simulink model "rpoco16"  (R2013a)
settings: Solver=VariableStepDiscrete  SolverMode=SingleTasking  StartTime=0.0  StopTime=10.0  RelTol=1e-3
libraries: xbsIndex_r4 x7152, casper_library_misc x156, casper_library_multipliers x68, casper_library_sources x8, xps_library x5, casper_library_delays x1
(part 9 of 84)

== system rpoco16/xengine16_muxed/bj ==
  a+bi : Inport
  c+di : Inport  Port=2
  new_acc : Inport  Port=3
  Convert{,1..3} (4 alike) : xbsIndex_r4/Convert  gui_display_data_type=Fixed-point  arith_type="Signed  (2's comp)"  n_bits=16  bin_pt=15  float_type=Single  exp_bits=8  fraction_bits=24  quantization="Round  (unbiased: Even Values)"  overflow=Wrap  en=off  latency=0  dbl_ovrd=off  pipeline=off  block_type=convert
      settings: block_version=11.4
  Counter2 : xbsIndex_r4/Counter  cnt_type=Free Running  cnt_to=Inf  operation=Up  start_count=0  cnt_by_val=1  arith_type=Unsigned  n_bits=max(nchan+1,11)  bin_pt=0  load_pin=off  rst=on  en=on  explicit_period=on  period=1  dbl_ovrd=off  use_behavioral_HDL=off  implementation=Fabric  use_rpm=off  block_type=counter
  Delay1 : xbsIndex_r4/Delay  rst=off  infoeditControl=Selection of Reset will increase slice count due to use of real FFs and instead of SRLs  en=off  latency=mult_latency + add_latency  dbl_ovrd=off  reg_retiming=off  block_type=delay
  c_to_ri : casper_library_misc/c_to_ri  n_bits=n_bits  bin_pt=n_bits-1
  c_to_ri1 : casper_library_misc/c_to_ri  n_bits=n_bits  bin_pt=n_bits-1
  cmult_4bit_em* : casper_library_multipliers/cmult_4bit_em*  mult_latency=mult_latency  add_latency=add_latency
  imag : Subsystem  Tag=xps:bram  AncestorBlock=xps_library/Shared BRAM  mask{arith_type=Signed  (2's comp), addr_width=max(nchan+1,11), data_width=32, reg_prim_output=off, reg_core_output=off, optimization=Minimum_Area, data_bin_pt=min(2*(n_bits-1), 30), init_vals=0, sample_rate=1}
      mask prompts: arith_type "Output Data Type"; addr_width "Address width"; data_width "Data Width"; reg_prim_output "Register Primitive Output"; reg_core_output "Register Core Output"; data_bin_pt "Data Binary Point"; init_vals "Initial values (simulation only)"; sample_rate "Sample rate"
      mask init:
      | shared_bram_mask;
      mask TypeOptions arith_type: Unsigned | Signed  (2's comp)
      mask TypeOptions data_width: 8 | 16 | 32 | 64 | 128
      mask TypeOptions optimization: Minimum_Area | Low_Power
  real : Subsystem  Tag=xps:bram  AncestorBlock=xps_library/Shared BRAM  mask{arith_type=Signed  (2's comp), addr_width=max(nchan+1,11), data_width=32, reg_prim_output=off, reg_core_output=off, optimization=Minimum_Area, data_bin_pt=min(2*(n_bits-1), 30), init_vals=0, sample_rate=1}
      mask prompts: arith_type "Output Data Type"; addr_width "Address width"; data_width "Data Width"; reg_prim_output "Register Primitive Output"; reg_core_output "Register Core Output"; data_bin_pt "Data Binary Point"; init_vals "Initial values (simulation only)"; sample_rate "Sample rate"
      mask init:
      | shared_bram_mask;
      mask TypeOptions arith_type: Unsigned | Signed  (2's comp)
      mask TypeOptions data_width: 8 | 16 | 32 | 64 | 128
      mask TypeOptions optimization: Minimum_Area | Low_Power
  simple_bram_vacc : Subsystem  AncestorBlock=casper_library_accumulators/simple_bram_vacc  mask(simple_bram_vacc){vec_len=2048, arith_type=Signed, n_bits=32, bin_pt=30}
      mask prompts: vec_len "Vector length:"; arith_type "Output type:"; n_bits "Bit width (output):"; bin_pt "Binary point (output):"
      mask help: This simple vector accumulator is based on a shift register. It outputs its previous accumulated vector after a new_acc pulse is received.
      mask init:
      | simple_bram_vacc_init(gcb, ...
      |     'vec_len', vec_len, ...
      |     'arith_type', arith_type, ...
      |     'n_bits', n_bits, ...
      |     'bin_pt', bin_pt);
      mask TypeOptions arith_type: Signed | Unsigned
  simple_bram_vacc1 : Subsystem  AncestorBlock=casper_library_accumulators/simple_bram_vacc  mask(simple_bram_vacc){vec_len=2048, arith_type=Signed, n_bits=32, bin_pt=30}
      mask prompts: vec_len "Vector length:"; arith_type "Output type:"; n_bits "Bit width (output):"; bin_pt "Binary point (output):"
      mask help: This simple vector accumulator is based on a shift register. It outputs its previous accumulated vector after a new_acc pulse is received.
      mask init:
      | simple_bram_vacc_init(gcb, ...
      |     'vec_len', vec_len, ...
      |     'arith_type', arith_type, ...
      |     'n_bits', n_bits, ...
      |     'bin_pt', bin_pt);
      mask TypeOptions arith_type: Signed | Unsigned
  wires:
  Convert3/1 -> cmult_4bit_em*/4
  Convert2/1 -> cmult_4bit_em*/3
  Convert1/1 -> cmult_4bit_em*/2
  Convert/1 -> cmult_4bit_em*/1
  c_to_ri/1 -> Convert/1
  c_to_ri/2 -> Convert1/1
  c_to_ri1/1 -> Convert2/1
  c_to_ri1/2 -> Convert3/1
  a+bi/1 -> c_to_ri/1
  c+di/1 -> c_to_ri1/1
  new_acc/1 -> Delay1/1
  simple_bram_vacc/2(valid) -> Counter2/2, real/3(we)
  Counter2/1 -> real/1(addr), imag/1(addr)
  simple_bram_vacc/1(dout) -> real/2(data_in)
  Delay1/1 -> simple_bram_vacc1/1(new_acc), simple_bram_vacc/1(new_acc), Counter2/1
  simple_bram_vacc1/1(dout) -> imag/2(data_in)
  simple_bram_vacc1/2(valid) -> imag/3(we)
  cmult_4bit_em*/1 -> simple_bram_vacc/2(din)
  cmult_4bit_em*/2 -> simple_bram_vacc1/2(din)

== system rpoco16/xengine16_muxed/bk ==
  a+bi : Inport
  c+di : Inport  Port=2
  new_acc : Inport  Port=3
  Convert{,1..3} (4 alike) : xbsIndex_r4/Convert  gui_display_data_type=Fixed-point  arith_type="Signed  (2's comp)"  n_bits=16  bin_pt=15  float_type=Single  exp_bits=8  fraction_bits=24  quantization="Round  (unbiased: Even Values)"  overflow=Wrap  en=off  latency=0  dbl_ovrd=off  pipeline=off  block_type=convert
      settings: block_version=11.4
  Counter2 : xbsIndex_r4/Counter  cnt_type=Free Running  cnt_to=Inf  operation=Up  start_count=0  cnt_by_val=1  arith_type=Unsigned  n_bits=max(nchan+1,11)  bin_pt=0  load_pin=off  rst=on  en=on  explicit_period=on  period=1  dbl_ovrd=off  use_behavioral_HDL=off  implementation=Fabric  use_rpm=off  block_type=counter
  Delay1 : xbsIndex_r4/Delay  rst=off  infoeditControl=Selection of Reset will increase slice count due to use of real FFs and instead of SRLs  en=off  latency=mult_latency + add_latency  dbl_ovrd=off  reg_retiming=off  block_type=delay
  c_to_ri : casper_library_misc/c_to_ri  n_bits=n_bits  bin_pt=n_bits-1
  c_to_ri1 : casper_library_misc/c_to_ri  n_bits=n_bits  bin_pt=n_bits-1
  cmult_4bit_em* : casper_library_multipliers/cmult_4bit_em*  mult_latency=mult_latency  add_latency=add_latency
  imag : Subsystem  Tag=xps:bram  AncestorBlock=xps_library/Shared BRAM  mask{arith_type=Signed  (2's comp), addr_width=max(nchan+1,11), data_width=32, reg_prim_output=off, reg_core_output=off, optimization=Minimum_Area, data_bin_pt=min(2*(n_bits-1), 30), init_vals=0, sample_rate=1}
      mask prompts: arith_type "Output Data Type"; addr_width "Address width"; data_width "Data Width"; reg_prim_output "Register Primitive Output"; reg_core_output "Register Core Output"; data_bin_pt "Data Binary Point"; init_vals "Initial values (simulation only)"; sample_rate "Sample rate"
      mask init:
      | shared_bram_mask;
      mask TypeOptions arith_type: Unsigned | Signed  (2's comp)
      mask TypeOptions data_width: 8 | 16 | 32 | 64 | 128
      mask TypeOptions optimization: Minimum_Area | Low_Power
  real : Subsystem  Tag=xps:bram  AncestorBlock=xps_library/Shared BRAM  mask{arith_type=Signed  (2's comp), addr_width=max(nchan+1,11), data_width=32, reg_prim_output=off, reg_core_output=off, optimization=Minimum_Area, data_bin_pt=min(2*(n_bits-1), 30), init_vals=0, sample_rate=1}
      mask prompts: arith_type "Output Data Type"; addr_width "Address width"; data_width "Data Width"; reg_prim_output "Register Primitive Output"; reg_core_output "Register Core Output"; data_bin_pt "Data Binary Point"; init_vals "Initial values (simulation only)"; sample_rate "Sample rate"
      mask init:
      | shared_bram_mask;
      mask TypeOptions arith_type: Unsigned | Signed  (2's comp)
      mask TypeOptions data_width: 8 | 16 | 32 | 64 | 128
      mask TypeOptions optimization: Minimum_Area | Low_Power
  simple_bram_vacc : Subsystem  AncestorBlock=casper_library_accumulators/simple_bram_vacc  mask(simple_bram_vacc){vec_len=2048, arith_type=Signed, n_bits=32, bin_pt=30}
      mask prompts: vec_len "Vector length:"; arith_type "Output type:"; n_bits "Bit width (output):"; bin_pt "Binary point (output):"
      mask help: This simple vector accumulator is based on a shift register. It outputs its previous accumulated vector after a new_acc pulse is received.
      mask init:
      | simple_bram_vacc_init(gcb, ...
      |     'vec_len', vec_len, ...
      |     'arith_type', arith_type, ...
      |     'n_bits', n_bits, ...
      |     'bin_pt', bin_pt);
      mask TypeOptions arith_type: Signed | Unsigned
  simple_bram_vacc1 : Subsystem  AncestorBlock=casper_library_accumulators/simple_bram_vacc  mask(simple_bram_vacc){vec_len=2048, arith_type=Signed, n_bits=32, bin_pt=30}
      mask prompts: vec_len "Vector length:"; arith_type "Output type:"; n_bits "Bit width (output):"; bin_pt "Binary point (output):"
      mask help: This simple vector accumulator is based on a shift register. It outputs its previous accumulated vector after a new_acc pulse is received.
      mask init:
      | simple_bram_vacc_init(gcb, ...
      |     'vec_len', vec_len, ...
      |     'arith_type', arith_type, ...
      |     'n_bits', n_bits, ...
      |     'bin_pt', bin_pt);
      mask TypeOptions arith_type: Signed | Unsigned
  wires:
  Convert3/1 -> cmult_4bit_em*/4
  Convert2/1 -> cmult_4bit_em*/3
  Convert1/1 -> cmult_4bit_em*/2
  Convert/1 -> cmult_4bit_em*/1
  c_to_ri/1 -> Convert/1
  c_to_ri/2 -> Convert1/1
  c_to_ri1/1 -> Convert2/1
  c_to_ri1/2 -> Convert3/1
  a+bi/1 -> c_to_ri/1
  c+di/1 -> c_to_ri1/1
  new_acc/1 -> Delay1/1
  simple_bram_vacc/2(valid) -> Counter2/2, real/3(we)
  Counter2/1 -> real/1(addr), imag/1(addr)
  simple_bram_vacc/1(dout) -> real/2(data_in)
  Delay1/1 -> simple_bram_vacc1/1(new_acc), simple_bram_vacc/1(new_acc), Counter2/1
  simple_bram_vacc1/1(dout) -> imag/2(data_in)
  simple_bram_vacc1/2(valid) -> imag/3(we)
  cmult_4bit_em*/1 -> simple_bram_vacc/2(din)
  cmult_4bit_em*/2 -> simple_bram_vacc1/2(din)

== system rpoco16/xengine16_muxed/bl ==
  a+bi : Inport
  c+di : Inport  Port=2
  new_acc : Inport  Port=3
  Convert{,1..3} (4 alike) : xbsIndex_r4/Convert  gui_display_data_type=Fixed-point  arith_type="Signed  (2's comp)"  n_bits=16  bin_pt=15  float_type=Single  exp_bits=8  fraction_bits=24  quantization="Round  (unbiased: Even Values)"  overflow=Wrap  en=off  latency=0  dbl_ovrd=off  pipeline=off  block_type=convert
      settings: block_version=11.4
  Counter2 : xbsIndex_r4/Counter  cnt_type=Free Running  cnt_to=Inf  operation=Up  start_count=0  cnt_by_val=1  arith_type=Unsigned  n_bits=max(nchan+1,11)  bin_pt=0  load_pin=off  rst=on  en=on  explicit_period=on  period=1  dbl_ovrd=off  use_behavioral_HDL=off  implementation=Fabric  use_rpm=off  block_type=counter
  Delay1 : xbsIndex_r4/Delay  rst=off  infoeditControl=Selection of Reset will increase slice count due to use of real FFs and instead of SRLs  en=off  latency=mult_latency + add_latency  dbl_ovrd=off  reg_retiming=off  block_type=delay
  c_to_ri : casper_library_misc/c_to_ri  n_bits=n_bits  bin_pt=n_bits-1
  c_to_ri1 : casper_library_misc/c_to_ri  n_bits=n_bits  bin_pt=n_bits-1
  cmult_4bit_em* : casper_library_multipliers/cmult_4bit_em*  mult_latency=mult_latency  add_latency=add_latency
  imag : Subsystem  Tag=xps:bram  AncestorBlock=xps_library/Shared BRAM  mask{arith_type=Signed  (2's comp), addr_width=max(nchan+1,11), data_width=32, reg_prim_output=off, reg_core_output=off, optimization=Minimum_Area, data_bin_pt=min(2*(n_bits-1), 30), init_vals=0, sample_rate=1}
      mask prompts: arith_type "Output Data Type"; addr_width "Address width"; data_width "Data Width"; reg_prim_output "Register Primitive Output"; reg_core_output "Register Core Output"; data_bin_pt "Data Binary Point"; init_vals "Initial values (simulation only)"; sample_rate "Sample rate"
      mask init:
      | shared_bram_mask;
      mask TypeOptions arith_type: Unsigned | Signed  (2's comp)
      mask TypeOptions data_width: 8 | 16 | 32 | 64 | 128
      mask TypeOptions optimization: Minimum_Area | Low_Power
  real : Subsystem  Tag=xps:bram  AncestorBlock=xps_library/Shared BRAM  mask{arith_type=Signed  (2's comp), addr_width=max(nchan+1,11), data_width=32, reg_prim_output=off, reg_core_output=off, optimization=Minimum_Area, data_bin_pt=min(2*(n_bits-1), 30), init_vals=0, sample_rate=1}
      mask prompts: arith_type "Output Data Type"; addr_width "Address width"; data_width "Data Width"; reg_prim_output "Register Primitive Output"; reg_core_output "Register Core Output"; data_bin_pt "Data Binary Point"; init_vals "Initial values (simulation only)"; sample_rate "Sample rate"
      mask init:
      | shared_bram_mask;
      mask TypeOptions arith_type: Unsigned | Signed  (2's comp)
      mask TypeOptions data_width: 8 | 16 | 32 | 64 | 128
      mask TypeOptions optimization: Minimum_Area | Low_Power
  simple_bram_vacc : Subsystem  AncestorBlock=casper_library_accumulators/simple_bram_vacc  mask(simple_bram_vacc){vec_len=2048, arith_type=Signed, n_bits=32, bin_pt=30}
      mask prompts: vec_len "Vector length:"; arith_type "Output type:"; n_bits "Bit width (output):"; bin_pt "Binary point (output):"
      mask help: This simple vector accumulator is based on a shift register. It outputs its previous accumulated vector after a new_acc pulse is received.
      mask init:
      | simple_bram_vacc_init(gcb, ...
      |     'vec_len', vec_len, ...
      |     'arith_type', arith_type, ...
      |     'n_bits', n_bits, ...
      |     'bin_pt', bin_pt);
      mask TypeOptions arith_type: Signed | Unsigned
  simple_bram_vacc1 : Subsystem  AncestorBlock=casper_library_accumulators/simple_bram_vacc  mask(simple_bram_vacc){vec_len=2048, arith_type=Signed, n_bits=32, bin_pt=30}
      mask prompts: vec_len "Vector length:"; arith_type "Output type:"; n_bits "Bit width (output):"; bin_pt "Binary point (output):"
      mask help: This simple vector accumulator is based on a shift register. It outputs its previous accumulated vector after a new_acc pulse is received.
      mask init:
      | simple_bram_vacc_init(gcb, ...
      |     'vec_len', vec_len, ...
      |     'arith_type', arith_type, ...
      |     'n_bits', n_bits, ...
      |     'bin_pt', bin_pt);
      mask TypeOptions arith_type: Signed | Unsigned
  wires:
  Convert3/1 -> cmult_4bit_em*/4
  Convert2/1 -> cmult_4bit_em*/3
  Convert1/1 -> cmult_4bit_em*/2
  Convert/1 -> cmult_4bit_em*/1
  c_to_ri/1 -> Convert/1
  c_to_ri/2 -> Convert1/1
  c_to_ri1/1 -> Convert2/1
  c_to_ri1/2 -> Convert3/1
  a+bi/1 -> c_to_ri/1
  c+di/1 -> c_to_ri1/1
  new_acc/1 -> Delay1/1
  simple_bram_vacc/2(valid) -> Counter2/2, real/3(we)
  Counter2/1 -> real/1(addr), imag/1(addr)
  simple_bram_vacc/1(dout) -> real/2(data_in)
  Delay1/1 -> simple_bram_vacc1/1(new_acc), simple_bram_vacc/1(new_acc), Counter2/1
  simple_bram_vacc1/1(dout) -> imag/2(data_in)
  simple_bram_vacc1/2(valid) -> imag/3(we)
  cmult_4bit_em*/1 -> simple_bram_vacc/2(din)
  cmult_4bit_em*/2 -> simple_bram_vacc1/2(din)

== system rpoco16/xengine16_muxed/cc ==
  a+bi : Inport
  c+di : Inport  Port=2
  new_acc : Inport  Port=3
  Convert{,1..3} (4 alike) : xbsIndex_r4/Convert  gui_display_data_type=Fixed-point  arith_type="Signed  (2's comp)"  n_bits=16  bin_pt=15  float_type=Single  exp_bits=8  fraction_bits=24  quantization="Round  (unbiased: Even Values)"  overflow=Wrap  en=off  latency=0  dbl_ovrd=off  pipeline=off  block_type=convert
      settings: block_version=11.4
  Counter2 : xbsIndex_r4/Counter  cnt_type=Free Running  cnt_to=Inf  operation=Up  start_count=0  cnt_by_val=1  arith_type=Unsigned  n_bits=max(nchan+1,11)  bin_pt=0  load_pin=off  rst=on  en=on  explicit_period=on  period=1  dbl_ovrd=off  use_behavioral_HDL=off  implementation=Fabric  use_rpm=off  block_type=counter
  Delay1 : xbsIndex_r4/Delay  rst=off  infoeditControl=Selection of Reset will increase slice count due to use of real FFs and instead of SRLs  en=off  latency=mult_latency + add_latency  dbl_ovrd=off  reg_retiming=off  block_type=delay
  c_to_ri : casper_library_misc/c_to_ri  n_bits=n_bits  bin_pt=n_bits-1
  c_to_ri1 : casper_library_misc/c_to_ri  n_bits=n_bits  bin_pt=n_bits-1
  cmult_4bit_em* : casper_library_multipliers/cmult_4bit_em*  mult_latency=mult_latency  add_latency=add_latency
  real : Subsystem  Tag=xps:bram  AncestorBlock=xps_library/Shared BRAM  mask{arith_type=Signed  (2's comp), addr_width=max(nchan+1,11), data_width=32, reg_prim_output=off, reg_core_output=off, optimization=Minimum_Area, data_bin_pt=min(2*(n_bits-1), 30), init_vals=0, sample_rate=1}
      mask prompts: arith_type "Output Data Type"; addr_width "Address width"; data_width "Data Width"; reg_prim_output "Register Primitive Output"; reg_core_output "Register Core Output"; data_bin_pt "Data Binary Point"; init_vals "Initial values (simulation only)"; sample_rate "Sample rate"
      mask init:
      | shared_bram_mask;
      mask TypeOptions arith_type: Unsigned | Signed  (2's comp)
      mask TypeOptions data_width: 8 | 16 | 32 | 64 | 128
      mask TypeOptions optimization: Minimum_Area | Low_Power
  simple_bram_vacc : Subsystem  AncestorBlock=casper_library_accumulators/simple_bram_vacc  mask(simple_bram_vacc){vec_len=2048, arith_type=Signed, n_bits=32, bin_pt=30}
      mask prompts: vec_len "Vector length:"; arith_type "Output type:"; n_bits "Bit width (output):"; bin_pt "Binary point (output):"
      mask help: This simple vector accumulator is based on a shift register. It outputs its previous accumulated vector after a new_acc pulse is received.
      mask init:
      | simple_bram_vacc_init(gcb, ...
      |     'vec_len', vec_len, ...
      |     'arith_type', arith_type, ...
      |     'n_bits', n_bits, ...
      |     'bin_pt', bin_pt);
      mask TypeOptions arith_type: Signed | Unsigned
  wires:
  cmult_4bit_em*/1 -> simple_bram_vacc/2(din)
  new_acc/1 -> Delay1/1
  c+di/1 -> c_to_ri1/1
  a+bi/1 -> c_to_ri/1
  simple_bram_vacc/2(valid) -> Counter2/2, real/3(we)
  Counter2/1 -> real/1(addr)
  simple_bram_vacc/1(dout) -> real/2(data_in)
  Delay1/1 -> Counter2/1, simple_bram_vacc/1(new_acc)
  c_to_ri1/2 -> Convert3/1
  c_to_ri1/1 -> Convert2/1
  c_to_ri/2 -> Convert1/1
  c_to_ri/1 -> Convert/1
  Convert/1 -> cmult_4bit_em*/1
  Convert1/1 -> cmult_4bit_em*/2
  Convert2/1 -> cmult_4bit_em*/3
  Convert3/1 -> cmult_4bit_em*/4

== system rpoco16/xengine16_muxed/cd ==
  a+bi : Inport
  c+di : Inport  Port=2
  new_acc : Inport  Port=3
  Convert{,1..3} (4 alike) : xbsIndex_r4/Convert  gui_display_data_type=Fixed-point  arith_type="Signed  (2's comp)"  n_bits=16  bin_pt=15  float_type=Single  exp_bits=8  fraction_bits=24  quantization="Round  (unbiased: Even Values)"  overflow=Wrap  en=off  latency=0  dbl_ovrd=off  pipeline=off  block_type=convert
      settings: block_version=11.4
  Counter2 : xbsIndex_r4/Counter  cnt_type=Free Running  cnt_to=Inf  operation=Up  start_count=0  cnt_by_val=1  arith_type=Unsigned  n_bits=max(nchan+1,11)  bin_pt=0  load_pin=off  rst=on  en=on  explicit_period=on  period=1  dbl_ovrd=off  use_behavioral_HDL=off  implementation=Fabric  use_rpm=off  block_type=counter
  Delay1 : xbsIndex_r4/Delay  rst=off  infoeditControl=Selection of Reset will increase slice count due to use of real FFs and instead of SRLs  en=off  latency=mult_latency + add_latency  dbl_ovrd=off  reg_retiming=off  block_type=delay
  c_to_ri : casper_library_misc/c_to_ri  n_bits=n_bits  bin_pt=n_bits-1
  c_to_ri1 : casper_library_misc/c_to_ri  n_bits=n_bits  bin_pt=n_bits-1
  cmult_4bit_em* : casper_library_multipliers/cmult_4bit_em*  mult_latency=mult_latency  add_latency=add_latency
  imag : Subsystem  Tag=xps:bram  AncestorBlock=xps_library/Shared BRAM  mask{arith_type=Signed  (2's comp), addr_width=max(nchan+1,11), data_width=32, reg_prim_output=off, reg_core_output=off, optimization=Minimum_Area, data_bin_pt=min(2*(n_bits-1), 30), init_vals=0, sample_rate=1}
      mask prompts: arith_type "Output Data Type"; addr_width "Address width"; data_width "Data Width"; reg_prim_output "Register Primitive Output"; reg_core_output "Register Core Output"; data_bin_pt "Data Binary Point"; init_vals "Initial values (simulation only)"; sample_rate "Sample rate"
      mask init:
      | shared_bram_mask;
      mask TypeOptions arith_type: Unsigned | Signed  (2's comp)
      mask TypeOptions data_width: 8 | 16 | 32 | 64 | 128
      mask TypeOptions optimization: Minimum_Area | Low_Power
  real : Subsystem  Tag=xps:bram  AncestorBlock=xps_library/Shared BRAM  mask{arith_type=Signed  (2's comp), addr_width=max(nchan+1,11), data_width=32, reg_prim_output=off, reg_core_output=off, optimization=Minimum_Area, data_bin_pt=min(2*(n_bits-1), 30), init_vals=0, sample_rate=1}
      mask prompts: arith_type "Output Data Type"; addr_width "Address width"; data_width "Data Width"; reg_prim_output "Register Primitive Output"; reg_core_output "Register Core Output"; data_bin_pt "Data Binary Point"; init_vals "Initial values (simulation only)"; sample_rate "Sample rate"
      mask init:
      | shared_bram_mask;
      mask TypeOptions arith_type: Unsigned | Signed  (2's comp)
      mask TypeOptions data_width: 8 | 16 | 32 | 64 | 128
      mask TypeOptions optimization: Minimum_Area | Low_Power
  simple_bram_vacc : Subsystem  AncestorBlock=casper_library_accumulators/simple_bram_vacc  mask(simple_bram_vacc){vec_len=2048, arith_type=Signed, n_bits=32, bin_pt=30}
      mask prompts: vec_len "Vector length:"; arith_type "Output type:"; n_bits "Bit width (output):"; bin_pt "Binary point (output):"
      mask help: This simple vector accumulator is based on a shift register. It outputs its previous accumulated vector after a new_acc pulse is received.
      mask init:
      | simple_bram_vacc_init(gcb, ...
      |     'vec_len', vec_len, ...
      |     'arith_type', arith_type, ...
      |     'n_bits', n_bits, ...
      |     'bin_pt', bin_pt);
      mask TypeOptions arith_type: Signed | Unsigned
  simple_bram_vacc1 : Subsystem  AncestorBlock=casper_library_accumulators/simple_bram_vacc  mask(simple_bram_vacc){vec_len=2048, arith_type=Signed, n_bits=32, bin_pt=30}
      mask prompts: vec_len "Vector length:"; arith_type "Output type:"; n_bits "Bit width (output):"; bin_pt "Binary point (output):"
      mask help: This simple vector accumulator is based on a shift register. It outputs its previous accumulated vector after a new_acc pulse is received.
      mask init:
      | simple_bram_vacc_init(gcb, ...
      |     'vec_len', vec_len, ...
      |     'arith_type', arith_type, ...
      |     'n_bits', n_bits, ...
      |     'bin_pt', bin_pt);
      mask TypeOptions arith_type: Signed | Unsigned
  wires:
  cmult_4bit_em*/2 -> simple_bram_vacc1/2(din)
  cmult_4bit_em*/1 -> simple_bram_vacc/2(din)
  simple_bram_vacc1/2(valid) -> imag/3(we)
  simple_bram_vacc1/1(dout) -> imag/2(data_in)
  Delay1/1 -> Counter2/1, simple_bram_vacc/1(new_acc), simple_bram_vacc1/1(new_acc)
  simple_bram_vacc/1(dout) -> real/2(data_in)
  Counter2/1 -> imag/1(addr), real/1(addr)
  simple_bram_vacc/2(valid) -> real/3(we), Counter2/2
  new_acc/1 -> Delay1/1
  c+di/1 -> c_to_ri1/1
  a+bi/1 -> c_to_ri/1
  c_to_ri1/2 -> Convert3/1
  c_to_ri1/1 -> Convert2/1
  c_to_ri/2 -> Convert1/1
  c_to_ri/1 -> Convert/1
  Convert/1 -> cmult_4bit_em*/1
  Convert1/1 -> cmult_4bit_em*/2
  Convert2/1 -> cmult_4bit_em*/3
  Convert3/1 -> cmult_4bit_em*/4

== system rpoco16/xengine16_muxed/ce ==
  a+bi : Inport
  c+di : Inport  Port=2
  new_acc : Inport  Port=3
  Convert{,1..3} (4 alike) : xbsIndex_r4/Convert  gui_display_data_type=Fixed-point  arith_type="Signed  (2's comp)"  n_bits=16  bin_pt=15  float_type=Single  exp_bits=8  fraction_bits=24  quantization="Round  (unbiased: Even Values)"  overflow=Wrap  en=off  latency=0  dbl_ovrd=off  pipeline=off  block_type=convert
      settings: block_version=11.4
  Counter2 : xbsIndex_r4/Counter  cnt_type=Free Running  cnt_to=Inf  operation=Up  start_count=0  cnt_by_val=1  arith_type=Unsigned  n_bits=max(nchan+1,11)  bin_pt=0  load_pin=off  rst=on  en=on  explicit_period=on  period=1  dbl_ovrd=off  use_behavioral_HDL=off  implementation=Fabric  use_rpm=off  block_type=counter
  Delay1 : xbsIndex_r4/Delay  rst=off  infoeditControl=Selection of Reset will increase slice count due to use of real FFs and instead of SRLs  en=off  latency=mult_latency + add_latency  dbl_ovrd=off  reg_retiming=off  block_type=delay
  c_to_ri : casper_library_misc/c_to_ri  n_bits=n_bits  bin_pt=n_bits-1
  c_to_ri1 : casper_library_misc/c_to_ri  n_bits=n_bits  bin_pt=n_bits-1
  cmult_4bit_em* : casper_library_multipliers/cmult_4bit_em*  mult_latency=mult_latency  add_latency=add_latency
  imag : Subsystem  Tag=xps:bram  AncestorBlock=xps_library/Shared BRAM  mask{arith_type=Signed  (2's comp), addr_width=max(nchan+1,11), data_width=32, reg_prim_output=off, reg_core_output=off, optimization=Minimum_Area, data_bin_pt=min(2*(n_bits-1), 30), init_vals=0, sample_rate=1}
      mask prompts: arith_type "Output Data Type"; addr_width "Address width"; data_width "Data Width"; reg_prim_output "Register Primitive Output"; reg_core_output "Register Core Output"; data_bin_pt "Data Binary Point"; init_vals "Initial values (simulation only)"; sample_rate "Sample rate"
      mask init:
      | shared_bram_mask;
      mask TypeOptions arith_type: Unsigned | Signed  (2's comp)
      mask TypeOptions data_width: 8 | 16 | 32 | 64 | 128
      mask TypeOptions optimization: Minimum_Area | Low_Power
  real : Subsystem  Tag=xps:bram  AncestorBlock=xps_library/Shared BRAM  mask{arith_type=Signed  (2's comp), addr_width=max(nchan+1,11), data_width=32, reg_prim_output=off, reg_core_output=off, optimization=Minimum_Area, data_bin_pt=min(2*(n_bits-1), 30), init_vals=0, sample_rate=1}
      mask prompts: arith_type "Output Data Type"; addr_width "Address width"; data_width "Data Width"; reg_prim_output "Register Primitive Output"; reg_core_output "Register Core Output"; data_bin_pt "Data Binary Point"; init_vals "Initial values (simulation only)"; sample_rate "Sample rate"
      mask init:
      | shared_bram_mask;
      mask TypeOptions arith_type: Unsigned | Signed  (2's comp)
      mask TypeOptions data_width: 8 | 16 | 32 | 64 | 128
      mask TypeOptions optimization: Minimum_Area | Low_Power
  simple_bram_vacc : Subsystem  AncestorBlock=casper_library_accumulators/simple_bram_vacc  mask(simple_bram_vacc){vec_len=2048, arith_type=Signed, n_bits=32, bin_pt=30}
      mask prompts: vec_len "Vector length:"; arith_type "Output type:"; n_bits "Bit width (output):"; bin_pt "Binary point (output):"
      mask help: This simple vector accumulator is based on a shift register. It outputs its previous accumulated vector after a new_acc pulse is received.
      mask init:
      | simple_bram_vacc_init(gcb, ...
      |     'vec_len', vec_len, ...
      |     'arith_type', arith_type, ...
      |     'n_bits', n_bits, ...
      |     'bin_pt', bin_pt);
      mask TypeOptions arith_type: Signed | Unsigned
  simple_bram_vacc1 : Subsystem  AncestorBlock=casper_library_accumulators/simple_bram_vacc  mask(simple_bram_vacc){vec_len=2048, arith_type=Signed, n_bits=32, bin_pt=30}
      mask prompts: vec_len "Vector length:"; arith_type "Output type:"; n_bits "Bit width (output):"; bin_pt "Binary point (output):"
      mask help: This simple vector accumulator is based on a shift register. It outputs its previous accumulated vector after a new_acc pulse is received.
      mask init:
      | simple_bram_vacc_init(gcb, ...
      |     'vec_len', vec_len, ...
      |     'arith_type', arith_type, ...
      |     'n_bits', n_bits, ...
      |     'bin_pt', bin_pt);
      mask TypeOptions arith_type: Signed | Unsigned
  wires:
  Convert3/1 -> cmult_4bit_em*/4
  Convert2/1 -> cmult_4bit_em*/3
  Convert1/1 -> cmult_4bit_em*/2
  Convert/1 -> cmult_4bit_em*/1
  c_to_ri/1 -> Convert/1
  c_to_ri/2 -> Convert1/1
  c_to_ri1/1 -> Convert2/1
  c_to_ri1/2 -> Convert3/1
  a+bi/1 -> c_to_ri/1
  c+di/1 -> c_to_ri1/1
  new_acc/1 -> Delay1/1
  simple_bram_vacc/2(valid) -> Counter2/2, real/3(we)
  Counter2/1 -> real/1(addr), imag/1(addr)
  simple_bram_vacc/1(dout) -> real/2(data_in)
  Delay1/1 -> simple_bram_vacc1/1(new_acc), simple_bram_vacc/1(new_acc), Counter2/1
  simple_bram_vacc1/1(dout) -> imag/2(data_in)
  simple_bram_vacc1/2(valid) -> imag/3(we)
  cmult_4bit_em*/1 -> simple_bram_vacc/2(din)
  cmult_4bit_em*/2 -> simple_bram_vacc1/2(din)

== system rpoco16/xengine16_muxed/cf ==
  a+bi : Inport
  c+di : Inport  Port=2
  new_acc : Inport  Port=3
  Convert{,1..3} (4 alike) : xbsIndex_r4/Convert  gui_display_data_type=Fixed-point  arith_type="Signed  (2's comp)"  n_bits=16  bin_pt=15  float_type=Single  exp_bits=8  fraction_bits=24  quantization="Round  (unbiased: Even Values)"  overflow=Wrap  en=off  latency=0  dbl_ovrd=off  pipeline=off  block_type=convert
      settings: block_version=11.4
  Counter2 : xbsIndex_r4/Counter  cnt_type=Free Running  cnt_to=Inf  operation=Up  start_count=0  cnt_by_val=1  arith_type=Unsigned  n_bits=max(nchan+1,11)  bin_pt=0  load_pin=off  rst=on  en=on  explicit_period=on  period=1  dbl_ovrd=off  use_behavioral_HDL=off  implementation=Fabric  use_rpm=off  block_type=counter
  Delay1 : xbsIndex_r4/Delay  rst=off  infoeditControl=Selection of Reset will increase slice count due to use of real FFs and instead of SRLs  en=off  latency=mult_latency + add_latency  dbl_ovrd=off  reg_retiming=off  block_type=delay
  c_to_ri : casper_library_misc/c_to_ri  n_bits=n_bits  bin_pt=n_bits-1
  c_to_ri1 : casper_library_misc/c_to_ri  n_bits=n_bits  bin_pt=n_bits-1
  cmult_4bit_em* : casper_library_multipliers/cmult_4bit_em*  mult_latency=mult_latency  add_latency=add_latency
  imag : Subsystem  Tag=xps:bram  AncestorBlock=xps_library/Shared BRAM  mask{arith_type=Signed  (2's comp), addr_width=max(nchan+1,11), data_width=32, reg_prim_output=off, reg_core_output=off, optimization=Minimum_Area, data_bin_pt=min(2*(n_bits-1), 30), init_vals=0, sample_rate=1}
      mask prompts: arith_type "Output Data Type"; addr_width "Address width"; data_width "Data Width"; reg_prim_output "Register Primitive Output"; reg_core_output "Register Core Output"; data_bin_pt "Data Binary Point"; init_vals "Initial values (simulation only)"; sample_rate "Sample rate"
      mask init:
      | shared_bram_mask;
      mask TypeOptions arith_type: Unsigned | Signed  (2's comp)
      mask TypeOptions data_width: 8 | 16 | 32 | 64 | 128
      mask TypeOptions optimization: Minimum_Area | Low_Power
  real : Subsystem  Tag=xps:bram  AncestorBlock=xps_library/Shared BRAM  mask{arith_type=Signed  (2's comp), addr_width=max(nchan+1,11), data_width=32, reg_prim_output=off, reg_core_output=off, optimization=Minimum_Area, data_bin_pt=min(2*(n_bits-1), 30), init_vals=0, sample_rate=1}
      mask prompts: arith_type "Output Data Type"; addr_width "Address width"; data_width "Data Width"; reg_prim_output "Register Primitive Output"; reg_core_output "Register Core Output"; data_bin_pt "Data Binary Point"; init_vals "Initial values (simulation only)"; sample_rate "Sample rate"
      mask init:
      | shared_bram_mask;
      mask TypeOptions arith_type: Unsigned | Signed  (2's comp)
      mask TypeOptions data_width: 8 | 16 | 32 | 64 | 128
      mask TypeOptions optimization: Minimum_Area | Low_Power
  simple_bram_vacc : Subsystem  AncestorBlock=casper_library_accumulators/simple_bram_vacc  mask(simple_bram_vacc){vec_len=2048, arith_type=Signed, n_bits=32, bin_pt=30}
      mask prompts: vec_len "Vector length:"; arith_type "Output type:"; n_bits "Bit width (output):"; bin_pt "Binary point (output):"
      mask help: This simple vector accumulator is based on a shift register. It outputs its previous accumulated vector after a new_acc pulse is received.
      mask init:
      | simple_bram_vacc_init(gcb, ...
      |     'vec_len', vec_len, ...
      |     'arith_type', arith_type, ...
      |     'n_bits', n_bits, ...
      |     'bin_pt', bin_pt);
      mask TypeOptions arith_type: Signed | Unsigned
  simple_bram_vacc1 : Subsystem  AncestorBlock=casper_library_accumulators/simple_bram_vacc  mask(simple_bram_vacc){vec_len=2048, arith_type=Signed, n_bits=32, bin_pt=30}
      mask prompts: vec_len "Vector length:"; arith_type "Output type:"; n_bits "Bit width (output):"; bin_pt "Binary point (output):"
      mask help: This simple vector accumulator is based on a shift register. It outputs its previous accumulated vector after a new_acc pulse is received.
      mask init:
      | simple_bram_vacc_init(gcb, ...
      |     'vec_len', vec_len, ...
      |     'arith_type', arith_type, ...
      |     'n_bits', n_bits, ...
      |     'bin_pt', bin_pt);
      mask TypeOptions arith_type: Signed | Unsigned
  wires:
  cmult_4bit_em*/2 -> simple_bram_vacc1/2(din)
  cmult_4bit_em*/1 -> simple_bram_vacc/2(din)
  simple_bram_vacc1/2(valid) -> imag/3(we)
  simple_bram_vacc1/1(dout) -> imag/2(data_in)
  Delay1/1 -> Counter2/1, simple_bram_vacc/1(new_acc), simple_bram_vacc1/1(new_acc)
  simple_bram_vacc/1(dout) -> real/2(data_in)
  Counter2/1 -> imag/1(addr), real/1(addr)
  simple_bram_vacc/2(valid) -> real/3(we), Counter2/2
  new_acc/1 -> Delay1/1
  c+di/1 -> c_to_ri1/1
  a+bi/1 -> c_to_ri/1
  c_to_ri1/2 -> Convert3/1
  c_to_ri1/1 -> Convert2/1
  c_to_ri/2 -> Convert1/1
  c_to_ri/1 -> Convert/1
  Convert/1 -> cmult_4bit_em*/1
  Convert1/1 -> cmult_4bit_em*/2
  Convert2/1 -> cmult_4bit_em*/3
  Convert3/1 -> cmult_4bit_em*/4

== system rpoco16/xengine16_muxed/cg ==
  a+bi : Inport
  c+di : Inport  Port=2
  new_acc : Inport  Port=3
  Convert{,1..3} (4 alike) : xbsIndex_r4/Convert  gui_display_data_type=Fixed-point  arith_type="Signed  (2's comp)"  n_bits=16  bin_pt=15  float_type=Single  exp_bits=8  fraction_bits=24  quantization="Round  (unbiased: Even Values)"  overflow=Wrap  en=off  latency=0  dbl_ovrd=off  pipeline=off  block_type=convert
      settings: block_version=11.4
  Counter2 : xbsIndex_r4/Counter  cnt_type=Free Running  cnt_to=Inf  operation=Up  start_count=0  cnt_by_val=1  arith_type=Unsigned  n_bits=max(nchan+1,11)  bin_pt=0  load_pin=off  rst=on  en=on  explicit_period=on  period=1  dbl_ovrd=off  use_behavioral_HDL=off  implementation=Fabric  use_rpm=off  block_type=counter
  Delay1 : xbsIndex_r4/Delay  rst=off  infoeditControl=Selection of Reset will increase slice count due to use of real FFs and instead of SRLs  en=off  latency=mult_latency + add_latency  dbl_ovrd=off  reg_retiming=off  block_type=delay
  c_to_ri : casper_library_misc/c_to_ri  n_bits=n_bits  bin_pt=n_bits-1
  c_to_ri1 : casper_library_misc/c_to_ri  n_bits=n_bits  bin_pt=n_bits-1
  cmult_4bit_em* : casper_library_multipliers/cmult_4bit_em*  mult_latency=mult_latency  add_latency=add_latency
  imag : Subsystem  Tag=xps:bram  AncestorBlock=xps_library/Shared BRAM  mask{arith_type=Signed  (2's comp), addr_width=max(nchan+1,11), data_width=32, reg_prim_output=off, reg_core_output=off, optimization=Minimum_Area, data_bin_pt=min(2*(n_bits-1), 30), init_vals=0, sample_rate=1}
      mask prompts: arith_type "Output Data Type"; addr_width "Address width"; data_width "Data Width"; reg_prim_output "Register Primitive Output"; reg_core_output "Register Core Output"; data_bin_pt "Data Binary Point"; init_vals "Initial values (simulation only)"; sample_rate "Sample rate"
      mask init:
      | shared_bram_mask;
      mask TypeOptions arith_type: Unsigned | Signed  (2's comp)
      mask TypeOptions data_width: 8 | 16 | 32 | 64 | 128
      mask TypeOptions optimization: Minimum_Area | Low_Power
  real : Subsystem  Tag=xps:bram  AncestorBlock=xps_library/Shared BRAM  mask{arith_type=Signed  (2's comp), addr_width=max(nchan+1,11), data_width=32, reg_prim_output=off, reg_core_output=off, optimization=Minimum_Area, data_bin_pt=min(2*(n_bits-1), 30), init_vals=0, sample_rate=1}
      mask prompts: arith_type "Output Data Type"; addr_width "Address width"; data_width "Data Width"; reg_prim_output "Register Primitive Output"; reg_core_output "Register Core Output"; data_bin_pt "Data Binary Point"; init_vals "Initial values (simulation only)"; sample_rate "Sample rate"
      mask init:
      | shared_bram_mask;
      mask TypeOptions arith_type: Unsigned | Signed  (2's comp)
      mask TypeOptions data_width: 8 | 16 | 32 | 64 | 128
      mask TypeOptions optimization: Minimum_Area | Low_Power
  simple_bram_vacc : Subsystem  AncestorBlock=casper_library_accumulators/simple_bram_vacc  mask(simple_bram_vacc){vec_len=2048, arith_type=Signed, n_bits=32, bin_pt=30}
      mask prompts: vec_len "Vector length:"; arith_type "Output type:"; n_bits "Bit width (output):"; bin_pt "Binary point (output):"
      mask help: This simple vector accumulator is based on a shift register. It outputs its previous accumulated vector after a new_acc pulse is received.
      mask init:
      | simple_bram_vacc_init(gcb, ...
      |     'vec_len', vec_len, ...
      |     'arith_type', arith_type, ...
      |     'n_bits', n_bits, ...
      |     'bin_pt', bin_pt);
      mask TypeOptions arith_type: Signed | Unsigned
  simple_bram_vacc1 : Subsystem  AncestorBlock=casper_library_accumulators/simple_bram_vacc  mask(simple_bram_vacc){vec_len=2048, arith_type=Signed, n_bits=32, bin_pt=30}
      mask prompts: vec_len "Vector length:"; arith_type "Output type:"; n_bits "Bit width (output):"; bin_pt "Binary point (output):"
      mask help: This simple vector accumulator is based on a shift register. It outputs its previous accumulated vector after a new_acc pulse is received.
      mask init:
      | simple_bram_vacc_init(gcb, ...
      |     'vec_len', vec_len, ...
      |     'arith_type', arith_type, ...
      |     'n_bits', n_bits, ...
      |     'bin_pt', bin_pt);
      mask TypeOptions arith_type: Signed | Unsigned
  wires:
  Convert3/1 -> cmult_4bit_em*/4
  Convert2/1 -> cmult_4bit_em*/3
  Convert1/1 -> cmult_4bit_em*/2
  Convert/1 -> cmult_4bit_em*/1
  c_to_ri/1 -> Convert/1
  c_to_ri/2 -> Convert1/1
  c_to_ri1/1 -> Convert2/1
  c_to_ri1/2 -> Convert3/1
  a+bi/1 -> c_to_ri/1
  c+di/1 -> c_to_ri1/1
  new_acc/1 -> Delay1/1
  simple_bram_vacc/2(valid) -> Counter2/2, real/3(we)
  Counter2/1 -> real/1(addr), imag/1(addr)
  simple_bram_vacc/1(dout) -> real/2(data_in)
  Delay1/1 -> simple_bram_vacc1/1(new_acc), simple_bram_vacc/1(new_acc), Counter2/1
  simple_bram_vacc1/1(dout) -> imag/2(data_in)
  simple_bram_vacc1/2(valid) -> imag/3(we)
  cmult_4bit_em*/1 -> simple_bram_vacc/2(din)
  cmult_4bit_em*/2 -> simple_bram_vacc1/2(din)

== system rpoco16/xengine16_muxed/ch ==
  a+bi : Inport
  c+di : Inport  Port=2
  new_acc : Inport  Port=3
  Convert{,1..3} (4 alike) : xbsIndex_r4/Convert  gui_display_data_type=Fixed-point  arith_type="Signed  (2's comp)"  n_bits=16  bin_pt=15  float_type=Single  exp_bits=8  fraction_bits=24  quantization="Round  (unbiased: Even Values)"  overflow=Wrap  en=off  latency=0  dbl_ovrd=off  pipeline=off  block_type=convert
      settings: block_version=11.4
  Counter2 : xbsIndex_r4/Counter  cnt_type=Free Running  cnt_to=Inf  operation=Up  start_count=0  cnt_by_val=1  arith_type=Unsigned  n_bits=max(nchan+1,11)  bin_pt=0  load_pin=off  rst=on  en=on  explicit_period=on  period=1  dbl_ovrd=off  use_behavioral_HDL=off  implementation=Fabric  use_rpm=off  block_type=counter
  Delay1 : xbsIndex_r4/Delay  rst=off  infoeditControl=Selection of Reset will increase slice count due to use of real FFs and instead of SRLs  en=off  latency=mult_latency + add_latency  dbl_ovrd=off  reg_retiming=off  block_type=delay
  c_to_ri : casper_library_misc/c_to_ri  n_bits=n_bits  bin_pt=n_bits-1
  c_to_ri1 : casper_library_misc/c_to_ri  n_bits=n_bits  bin_pt=n_bits-1
  cmult_4bit_em* : casper_library_multipliers/cmult_4bit_em*  mult_latency=mult_latency  add_latency=add_latency
  imag : Subsystem  Tag=xps:bram  AncestorBlock=xps_library/Shared BRAM  mask{arith_type=Signed  (2's comp), addr_width=max(nchan+1,11), data_width=32, reg_prim_output=off, reg_core_output=off, optimization=Minimum_Area, data_bin_pt=min(2*(n_bits-1), 30), init_vals=0, sample_rate=1}
      mask prompts: arith_type "Output Data Type"; addr_width "Address width"; data_width "Data Width"; reg_prim_output "Register Primitive Output"; reg_core_output "Register Core Output"; data_bin_pt "Data Binary Point"; init_vals "Initial values (simulation only)"; sample_rate "Sample rate"
      mask init:
      | shared_bram_mask;
      mask TypeOptions arith_type: Unsigned | Signed  (2's comp)
      mask TypeOptions data_width: 8 | 16 | 32 | 64 | 128
      mask TypeOptions optimization: Minimum_Area | Low_Power
  real : Subsystem  Tag=xps:bram  AncestorBlock=xps_library/Shared BRAM  mask{arith_type=Signed  (2's comp), addr_width=max(nchan+1,11), data_width=32, reg_prim_output=off, reg_core_output=off, optimization=Minimum_Area, data_bin_pt=min(2*(n_bits-1), 30), init_vals=0, sample_rate=1}
      mask prompts: arith_type "Output Data Type"; addr_width "Address width"; data_width "Data Width"; reg_prim_output "Register Primitive Output"; reg_core_output "Register Core Output"; data_bin_pt "Data Binary Point"; init_vals "Initial values (simulation only)"; sample_rate "Sample rate"
      mask init:
      | shared_bram_mask;
      mask TypeOptions arith_type: Unsigned | Signed  (2's comp)
      mask TypeOptions data_width: 8 | 16 | 32 | 64 | 128
      mask TypeOptions optimization: Minimum_Area | Low_Power
  simple_bram_vacc : Subsystem  AncestorBlock=casper_library_accumulators/simple_bram_vacc  mask(simple_bram_vacc){vec_len=2048, arith_type=Signed, n_bits=32, bin_pt=30}
      mask prompts: vec_len "Vector length:"; arith_type "Output type:"; n_bits "Bit width (output):"; bin_pt "Binary point (output):"
      mask help: This simple vector accumulator is based on a shift register. It outputs its previous accumulated vector after a new_acc pulse is received.
      mask init:
      | simple_bram_vacc_init(gcb, ...
      |     'vec_len', vec_len, ...
      |     'arith_type', arith_type, ...
      |     'n_bits', n_bits, ...
      |     'bin_pt', bin_pt);
      mask TypeOptions arith_type: Signed | Unsigned
  simple_bram_vacc1 : Subsystem  AncestorBlock=casper_library_accumulators/simple_bram_vacc  mask(simple_bram_vacc){vec_len=2048, arith_type=Signed, n_bits=32, bin_pt=30}
      mask prompts: vec_len "Vector length:"; arith_type "Output type:"; n_bits "Bit width (output):"; bin_pt "Binary point (output):"
      mask help: This simple vector accumulator is based on a shift register. It outputs its previous accumulated vector after a new_acc pulse is received.
      mask init:
      | simple_bram_vacc_init(gcb, ...
      |     'vec_len', vec_len, ...
      |     'arith_type', arith_type, ...
      |     'n_bits', n_bits, ...
      |     'bin_pt', bin_pt);
      mask TypeOptions arith_type: Signed | Unsigned
  wires:
  cmult_4bit_em*/2 -> simple_bram_vacc1/2(din)
  cmult_4bit_em*/1 -> simple_bram_vacc/2(din)
  simple_bram_vacc1/2(valid) -> imag/3(we)
  simple_bram_vacc1/1(dout) -> imag/2(data_in)
  Delay1/1 -> Counter2/1, simple_bram_vacc/1(new_acc), simple_bram_vacc1/1(new_acc)
  simple_bram_vacc/1(dout) -> real/2(data_in)
  Counter2/1 -> imag/1(addr), real/1(addr)
  simple_bram_vacc/2(valid) -> real/3(we), Counter2/2
  new_acc/1 -> Delay1/1
  c+di/1 -> c_to_ri1/1
  a+bi/1 -> c_to_ri/1
  c_to_ri1/2 -> Convert3/1
  c_to_ri1/1 -> Convert2/1
  c_to_ri/2 -> Convert1/1
  c_to_ri/1 -> Convert/1
  Convert/1 -> cmult_4bit_em*/1
  Convert1/1 -> cmult_4bit_em*/2
  Convert2/1 -> cmult_4bit_em*/3
  Convert3/1 -> cmult_4bit_em*/4

== system rpoco16/xengine16_muxed/ci ==
  a+bi : Inport
  c+di : Inport  Port=2
  new_acc : Inport  Port=3
  Convert{,1..3} (4 alike) : xbsIndex_r4/Convert  gui_display_data_type=Fixed-point  arith_type="Signed  (2's comp)"  n_bits=16  bin_pt=15  float_type=Single  exp_bits=8  fraction_bits=24  quantization="Round  (unbiased: Even Values)"  overflow=Wrap  en=off  latency=0  dbl_ovrd=off  pipeline=off  block_type=convert
      settings: block_version=11.4
  Counter2 : xbsIndex_r4/Counter  cnt_type=Free Running  cnt_to=Inf  operation=Up  start_count=0  cnt_by_val=1  arith_type=Unsigned  n_bits=max(nchan+1,11)  bin_pt=0  load_pin=off  rst=on  en=on  explicit_period=on  period=1  dbl_ovrd=off  use_behavioral_HDL=off  implementation=Fabric  use_rpm=off  block_type=counter
  Delay1 : xbsIndex_r4/Delay  rst=off  infoeditControl=Selection of Reset will increase slice count due to use of real FFs and instead of SRLs  en=off  latency=mult_latency + add_latency  dbl_ovrd=off  reg_retiming=off  block_type=delay
  c_to_ri : casper_library_misc/c_to_ri  n_bits=n_bits  bin_pt=n_bits-1
  c_to_ri1 : casper_library_misc/c_to_ri  n_bits=n_bits  bin_pt=n_bits-1
  cmult_4bit_em* : casper_library_multipliers/cmult_4bit_em*  mult_latency=mult_latency  add_latency=add_latency
  imag : Subsystem  Tag=xps:bram  AncestorBlock=xps_library/Shared BRAM  mask{arith_type=Signed  (2's comp), addr_width=max(nchan+1,11), data_width=32, reg_prim_output=off, reg_core_output=off, optimization=Minimum_Area, data_bin_pt=min(2*(n_bits-1), 30), init_vals=0, sample_rate=1}
      mask prompts: arith_type "Output Data Type"; addr_width "Address width"; data_width "Data Width"; reg_prim_output "Register Primitive Output"; reg_core_output "Register Core Output"; data_bin_pt "Data Binary Point"; init_vals "Initial values (simulation only)"; sample_rate "Sample rate"
      mask init:
      | shared_bram_mask;
      mask TypeOptions arith_type: Unsigned | Signed  (2's comp)
      mask TypeOptions data_width: 8 | 16 | 32 | 64 | 128
      mask TypeOptions optimization: Minimum_Area | Low_Power
  real : Subsystem  Tag=xps:bram  AncestorBlock=xps_library/Shared BRAM  mask{arith_type=Signed  (2's comp), addr_width=max(nchan+1,11), data_width=32, reg_prim_output=off, reg_core_output=off, optimization=Minimum_Area, data_bin_pt=min(2*(n_bits-1), 30), init_vals=0, sample_rate=1}
      mask prompts: arith_type "Output Data Type"; addr_width "Address width"; data_width "Data Width"; reg_prim_output "Register Primitive Output"; reg_core_output "Register Core Output"; data_bin_pt "Data Binary Point"; init_vals "Initial values (simulation only)"; sample_rate "Sample rate"
      mask init:
      | shared_bram_mask;
      mask TypeOptions arith_type: Unsigned | Signed  (2's comp)
      mask TypeOptions data_width: 8 | 16 | 32 | 64 | 128
      mask TypeOptions optimization: Minimum_Area | Low_Power
  simple_bram_vacc : Subsystem  AncestorBlock=casper_library_accumulators/simple_bram_vacc  mask(simple_bram_vacc){vec_len=2048, arith_type=Signed, n_bits=32, bin_pt=30}
      mask prompts: vec_len "Vector length:"; arith_type "Output type:"; n_bits "Bit width (output):"; bin_pt "Binary point (output):"
      mask help: This simple vector accumulator is based on a shift register. It outputs its previous accumulated vector after a new_acc pulse is received.
      mask init:
      | simple_bram_vacc_init(gcb, ...
      |     'vec_len', vec_len, ...
      |     'arith_type', arith_type, ...
      |     'n_bits', n_bits, ...
      |     'bin_pt', bin_pt);
      mask TypeOptions arith_type: Signed | Unsigned
  simple_bram_vacc1 : Subsystem  AncestorBlock=casper_library_accumulators/simple_bram_vacc  mask(simple_bram_vacc){vec_len=2048, arith_type=Signed, n_bits=32, bin_pt=30}
      mask prompts: vec_len "Vector length:"; arith_type "Output type:"; n_bits "Bit width (output):"; bin_pt "Binary point (output):"
      mask help: This simple vector accumulator is based on a shift register. It outputs its previous accumulated vector after a new_acc pulse is received.
      mask init:
      | simple_bram_vacc_init(gcb, ...
      |     'vec_len', vec_len, ...
      |     'arith_type', arith_type, ...
      |     'n_bits', n_bits, ...
      |     'bin_pt', bin_pt);
      mask TypeOptions arith_type: Signed | Unsigned
  wires:
  Convert3/1 -> cmult_4bit_em*/4
  Convert2/1 -> cmult_4bit_em*/3
  Convert1/1 -> cmult_4bit_em*/2
  Convert/1 -> cmult_4bit_em*/1
  c_to_ri/1 -> Convert/1
  c_to_ri/2 -> Convert1/1
  c_to_ri1/1 -> Convert2/1
  c_to_ri1/2 -> Convert3/1
  a+bi/1 -> c_to_ri/1
  c+di/1 -> c_to_ri1/1
  new_acc/1 -> Delay1/1
  simple_bram_vacc/2(valid) -> Counter2/2, real/3(we)
  Counter2/1 -> real/1(addr), imag/1(addr)
  simple_bram_vacc/1(dout) -> real/2(data_in)
  Delay1/1 -> simple_bram_vacc1/1(new_acc), simple_bram_vacc/1(new_acc), Counter2/1
  simple_bram_vacc1/1(dout) -> imag/2(data_in)
  simple_bram_vacc1/2(valid) -> imag/3(we)
  cmult_4bit_em*/1 -> simple_bram_vacc/2(din)
  cmult_4bit_em*/2 -> simple_bram_vacc1/2(din)
